simulink model "AGVsTrajectory"  (R2019b)
settings: Solver=VariableStepAuto  StartTime=0.0  StopTime=250  RelTol=1e-3
libraries: robotmobilelib x2
settings Model: PacingRate=3  Creator=Khaled  LastModifiedBy=Khaled

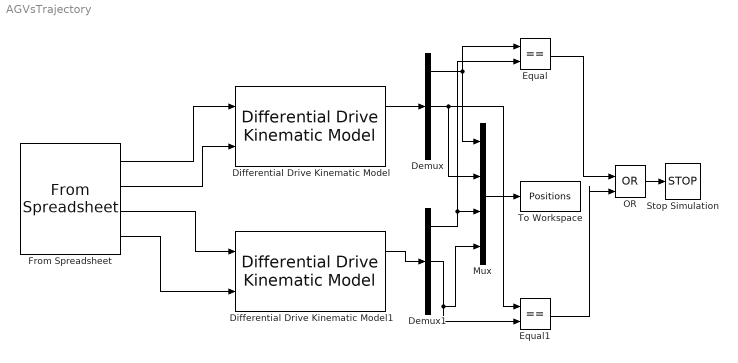
== system AGVsTrajectory ==
  Demux : Demux  Outputs=3
  Demux1 : Demux  Outputs=3
  Differential Drive Kinematic Model : robotmobilelib/Differential Drive Kinematic Model  VehicleInputs=Vehicle Speed & Heading Angular Velocity  WheelRadius=0.01  WheelSpeedRange=[-inf inf]  TrackWidth=0.15  InitialState=[0.8; 0.5; 0.655043]  SimulateUsing=Code generation
      settings: SourceProductName=Robotics System Toolbox  SourceProductBaseCode=RO
  Differential Drive Kinematic Model1 : robotmobilelib/Differential Drive Kinematic Model  VehicleInputs=Vehicle Speed & Heading Angular Velocity  WheelRadius=0.01  WheelSpeedRange=[-inf inf]  TrackWidth=0.15  InitialState=[1.13; 0.4; -0.13643]  SimulateUsing=Code generation
      settings: SourceProductName=Robotics System Toolbox  SourceProductBaseCode=RO
  Equal : RelationalOperator  Operator===  OutDataTypeStr=boolean  RndMeth=Simplest
  Equal1 : RelationalOperator  Operator===  OutDataTypeStr=boolean  RndMeth=Simplest
  From Spreadsheet : FromSpreadsheet  FileName=AGVs.xlsx  SheetName=Sheet2  SampleTime=-1
      mask Display: image('C:\Users\Khaled\Desktop\macos-app-icons-microsoft-excel-png-icon.jpg'); % Use "Edit Image" on toolstrip to change.
  Mux : Mux
  OR : Logic  Operator=OR  IconShape=distinctive  AllPortsSameDT=off  OutDataTypeStr=boolean
  Stop Simulation : Stop
  To Workspace : ToWorkspace  VariableName=Positions  SampleTime=0.1
  wires:
  Mux/1 -> To Workspace/1
  From Spreadsheet/3 -> Differential Drive Kinematic Model1/1
  Differential Drive Kinematic Model1/1 -> Demux1/1
  Demux1/1 -> Equal/2, Mux/3
  From Spreadsheet/4 -> Differential Drive Kinematic Model1/2
  From Spreadsheet/2 -> Differential Drive Kinematic Model/2
  Demux/1 -> Mux/1, Equal/1
  Demux1/2 -> Equal1/2, Mux/4
  Demux/2 -> Equal1/1, Mux/2
  From Spreadsheet/1 -> Differential Drive Kinematic Model/1
  Differential Drive Kinematic Model/1 -> Demux/1
  Equal/1 -> OR/1
  Equal1/1 -> OR/2
  OR/1 -> Stop Simulation/1
